simulink model "endmagsys"  (R2019b)
settings: Solver=VariableStepAuto  StartTime=0.0  StopTime=10.0  RelTol=1e-3
settings Model: Creator=Hamidreza  LastModifiedBy=Hamidreza

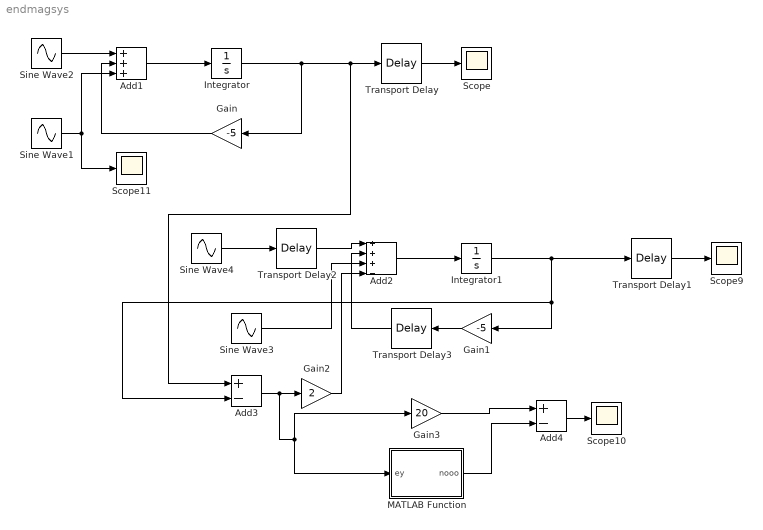
== system endmagsys ==
  Add1 : Sum  Inputs=+++
  Add2 : Sum  Inputs=+++-
  Add3 : Sum  Inputs=+-
  Add4 : Sum  Inputs=+-
  Gain : Gain  Gain=-5
  Gain1 : Gain  Gain=-5
  Gain2 : Gain  Gain=2
  Gain3 : Gain  Gain=20
  Integrator : Integrator
  Integrator1 : Integrator
  MATLAB Function : MATLAB Function  TreatAsAtomicUnit=on
  Scope{,9..11} (4 alike) : Scope
  Sine Wave1 : Sin  Amplitude=0.6  Frequency=2  SampleTime=0
  Sine Wave2 : Sin  Frequency=2  SampleTime=0
  Sine Wave3 : Sin  Amplitude=0.6  Frequency=2  SampleTime=0
  Sine Wave4 : Sin  Frequency=2  SampleTime=0
  Transport Delay{,1..3} (4 alike) : TransportDelay  DelayTime=0.1
  wires:
  Add4/1 -> Scope10/1
  Integrator1/1 -> Add3/2, Gain1/1, Transport Delay1/1
  Gain1/1 -> Transport Delay3/1
  Add2/1 -> Integrator1/1
  MATLAB Function/1(nooo) -> Add4/2
  Transport Delay/1 -> Scope/1
  Sine Wave4/1 -> Transport Delay2/1
  Sine Wave2/1 -> Add1/1
  Gain3/1 -> Add4/1
  Gain2/1 -> Add2/4
  Integrator/1 -> Gain/1, Add3/1, Transport Delay/1
  Sine Wave3/1 -> Add2/3
  Transport Delay3/1 -> Add2/2
  Add1/1 -> Integrator/1
  Transport Delay1/1 -> Scope9/1
  Add3/1 -> MATLAB Function/1(ey), Gain3/1, Gain2/1
  Sine Wave1/1 -> Scope11/1, Add1/3
  Transport Delay2/1 -> Add2/1
  Gain/1 -> Add1/2

== matlab function endmagsys/MATLAB Function ==
  data: ey input; nooo output
function nooo = fcn(ey)

nooo=(-2*ey)/(norm(ey)+0.01);
